simulink model "evitaparedes"  (R2023b)
settings: Solver=VariableStepAuto  StartTime=0.0  StopTime=10.0  RelTol=1e-3  EnableMultiTasking=on
settings Model: ExtModeTrigDuration=2  Creator=Usuario  LastModifiedBy=Usuario
settings RTWCC: BuildConfiguration=Faster Runs

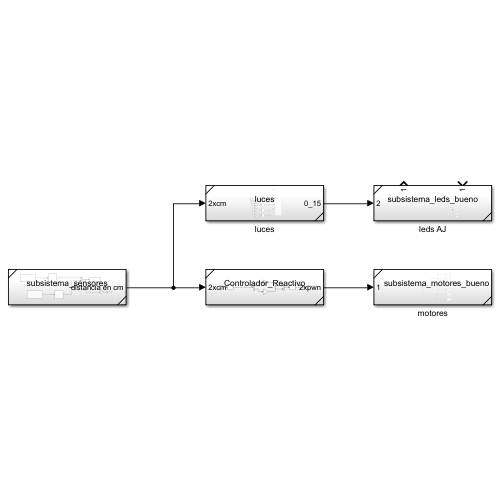
[thumbnail: Simulink's stored preview of the top-level diagram]
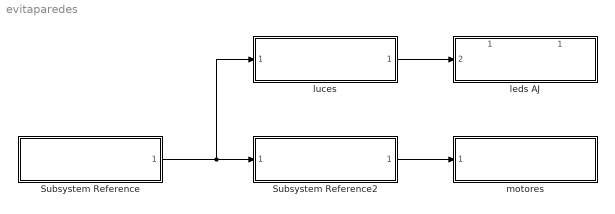
== system evitaparedes ==
  Subsystem Reference : Subsystem  ReferencedSubsystem=subsistema_sensores
  Subsystem Reference2 : Subsystem  ReferencedSubsystem=Controlador_Reactivo
  leds AJ : Subsystem  ReferencedSubsystem=subsistema_leds_bueno
      settings: PortSchema="{\"entries\":[{\"content\":{\"sides\":[{\"content\":{\"connectorIds\":[\"In2\"]},\"type\":\"ConnectorPlacement.EquallySpacedRectSide\",\"uuid\":\"de97dbf3-cdc3-422a-9c13-6e83e47795e5\"},{\"content\":{\"side\":\"RIGHT\"},\"type\":\"ConnectorPlacement.EquallySpacedRectSide\",\"uuid\":\"8cf22142-8993-41b1-a4d6-2412ad5159fc\"},{\"content\":{\"connectorIds\":[\"Out1\",\"In1\"],\"side\":\"TOP\"},\"type\":\"ConnectorPlacement.EquallySpacedRectSide\",\"uuid\":\"a0bec253-1ab2-4bc2-9a97-5efe4297aa62\"}]},\"type\":\"ConnectorPlacement.EquallySpacedConnector\",\"uuid\":\"ccffde28-9705-4e8a-98e3-d8587c6005c8\"}],\"packageUris\":[\"http://schema.mathworks.com/mf0/Connector/R2020b\"],\"version\":\"1.0\"}"
  luces : Subsystem  ReferencedSubsystem=luces
  motores : Subsystem  ReferencedSubsystem=subsistema_motores_bueno
  wires:
  Subsystem Reference/1 -> luces/1, Subsystem Reference2/1
  Subsystem Reference2/1 -> motores/1
  luces/1 -> leds AJ/2
